simulink model "testEmplanner_cs"  (R2021b)
settings: Solver=ode5  StartTime=0.0  StopTime=60  FixedStep=1/1000  RelTol=1e-3
PreLoadFcn:
  | mbxruntime.callbacks.PreLoadFcn(bdroot);
PostLoadFcn:
  | mbxruntime.callbacks.PostLoadFcn(bdroot);
InitFcn:
  | mbxruntime.callbacks.InitFcn(bdroot);
StartFcn:
  | mbxruntime.callbacks.StartFcn(bdroot);
StopFcn:
  | mbxruntime.callbacks.StopFcn(bdroot);
model workspace (MAT data in the model file):
  mbox_table : object (value not decoded)
  model_closed = 0
  sim_status = 0
values from neighbouring files (symbols this model uses):
  c_factor = 43.75    [emplanner_init.m]
  cf = -175016    [emplanner_init.m]
  cr = -130634    [emplanner_init.m]
  global_path_x = [-1.1448 -0.145417744933 0.852705365581 1.84955224935 2.84511712279 3.83939835808 4.83239585569 5.82411007764 6.81454169183 7.80369144113 8.79156009523 9.77814843293 ... (3001 elements, 3001x1)]    [global_path.mat]
  global_path_y = [14.6488 14.6488 14.6488 14.6488 14.6488 14.6488 14.6488 14.6488 14.6488 14.6488 14.6488 14.6488 ... (3001 elements, 3001x1)]    [global_path.mat]
  KD_PID_distance = 0.0    (= 0)    [emplanner_init.m]
  KD_PID_speed = 0    [emplanner_init.m]
  KI_PID_distance = 0.0    (= 0)    [emplanner_init.m]
  KI_PID_speed = 0    [emplanner_init.m]
  KP_PID_distance = 0.5    [emplanner_init.m]
  KP_PID_speed = 1.8    [emplanner_init.m]
  la = 1.265    [emplanner_init.m]
  lb = 2.947-1.265    (= 1.682)    [emplanner_init.m]
  LQR_K1 = k(:,1)'    [emplanner_init.m]
  LQR_K2 = k(:,2)'    [emplanner_init.m]
  LQR_K3 = k(:,3)'    [emplanner_init.m]
  LQR_K4 = k(:,4)'    [emplanner_init.m]
  m = 2020    [emplanner_init.m]
  rack_displacement = [-39.14 , -37.2 , -35.29 , -33.43 , -31.6 , -29.81 , -28.06 , -26.34 , -24.66 ,      -23.01 , -21.38 , -19.79 , -18.23 , -16.69 , -15.18 , -13.7 , -12.23 , -10.8 , -9.38 , -7.98 ,     -6.61 , -5.25 , -3.91 , -2.59 , -1.29 , 0 , 1.27 , 2.54 , 3.78 , 5.02 , 6.24 , 7.46 , 8.66 ,      9.86 , 11.05 , 12.24 , 13.41 , 14.59 , 15.76 , 16.92 , 18.09 , 19.25 , 20.42 , 21.59 , 22.76 ,      23.93 , 25.11 , 26 ...(+26 chars)    [emplanner_init.m]
  right_wheel_ground = [-70 ,-67.2 , -64.4 , -61.6 , -58.8 , -56 , -53.2 , -50.4 , -47.6 , -44.8 , -42 ,      -39.2 , -36.4 , -33.6 , -30.8 , -28 , -25.2 , -22.4 , -19.6 , -16.8 , -14 , -11.2 , -8.4 , -5.6 ,      -2.8 , 0 , 2.8 , 5.6 , 8.4 , 11.2 , 14 , 16.8 , 19.6 , 22.4 , 25.2 , 28 , 30.8 , 33.6 , 36.4 ,      39.2 , 42 , 44.8 , 47.6 , 50.4 , 53.2 , 56 , 58.8 , 61.6 , 64.4 , 67.2 , 70 ]    [emplanner_init.m]
  vx_break_point = zeros(1,5000)    [emplanner_init.m]
undefined symbols (not defined in the file or in its folder): aubr, DiscIntNeverNeededParam, tablebr, vubr, warningInitialVelocity, x0
libraries: simulink x19, PreScanSimulinkLibrary x17, simulink_extras x6, Solver_SF x1
(part 4 of 14)

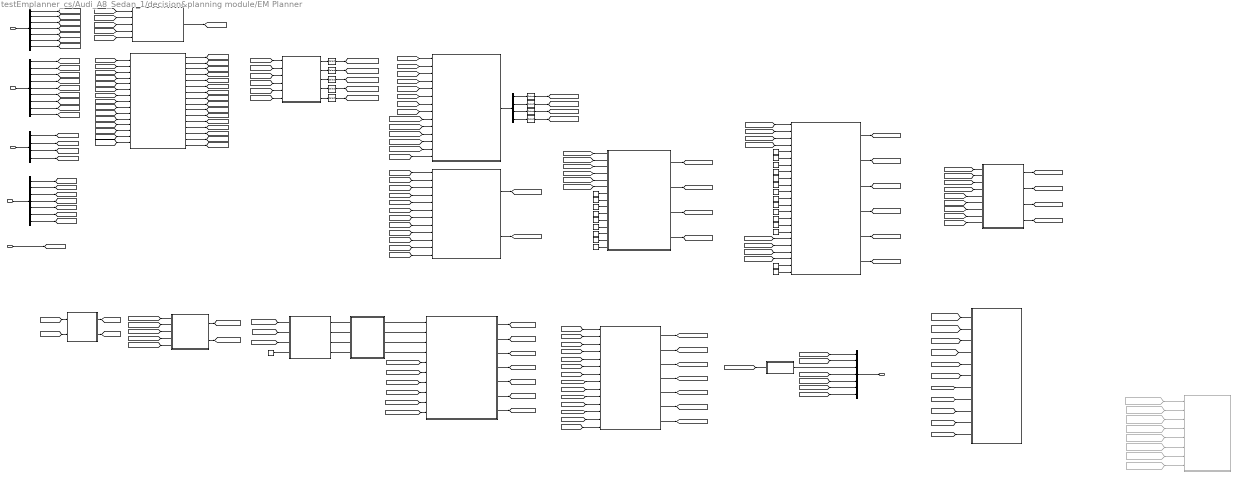
== system testEmplanner_cs/Audi_A8_Sedan_1/decision&planning module/EM Planner ==
  referenceline info : Inport
  location info : Inport  Port=2
  perception info : Inport  Port=3
  pre_planning info : Inport  Port=4
  current time : Inport  Port=5
  Bus Creator : BusCreator  Inputs=7
  Bus Selector : BusSelector  OutputSignals=host_x,host_y,host_heading_xy,host_vx,host_vy,host_yawrate,host_speed,host_ax,host_ay
  Bus Selector1 : BusSelector  OutputSignals=referenceline_x,referenceline_y,referenceline_heading,referenceline_kappa,origin_match_point_index,origin_x,origin_y
  Bus Selector2 : BusSelector  OutputSignals=obs_x_set_gcs,obs_y_set_gcs,obs_velocity_set_gcs,obs_heading_set_gcs
  Bus Selector3 : BusSelector  OutputSignals=trajectory_x_gcs,trajectory_y_gcs,trajectory_heading_gcs,trajectory_kappa_gcs,trajectory_speed_gcs,trajectory_accel_gcs,trajectory_time_gcs
  Bus Selector4 : BusSelector  OutputSignals=s_set,l_set,dl_set,ddl_set
  Cartesian2Frenet : Subsystem
  Constant : Constant  Value=1e8
  Constant1 : Constant  Value=300
  Constant10 : Constant  Value=5
  Constant11 : Constant  Value=2
  Constant12 : Constant  Value=0.1
  Constant13 : Constant  Value=0.02
  Constant14 : Constant  Value=2
  Constant15 : Constant  Value=25000
  Constant16 : Constant  Value=50
  Constant17 : Constant  Value=20
  Constant18 : Constant  Value=40
  Constant{7,19..21} (4 alike) : Constant  Value=15
  Constant2 : Constant  Value=10000
  Constant22 : Constant  Value=3
  Constant23 : Constant  Value=3
  Constant25 : Constant  Value=1.63
  Constant3 : Constant  Value=2000
  Constant4 : Constant  Value=20
  Constant5 : Constant  Value=9
  Constant6 : Constant  Value=4
  Constant8 : Constant
  Constant9 : Constant  Value=6
  Frenet2Cartesian : MATLAB Function  TreatAsAtomicUnit=on
  From165 : From  Commented=on  GotoTag=obs_st_s_in_set
  From166 : From  Commented=on  GotoTag=obs_st_s_out_set
  From167 : From  Commented=on  GotoTag=obs_st_t_in_set
  From168 : From  Commented=on  GotoTag=obs_st_t_out_set
  From177 : From  Commented=on  GotoTag=qp_s_init
  From178 : From  Commented=on  GotoTag=relative_time_init
  From90 : From  Commented=on  GotoTag=dp_speed_s
  From91 : From  Commented=on  GotoTag=dp_speed_t
  MATLAB Function : MATLAB Function  TreatAsAtomicUnit=on
  MATLAB Function3 : MATLAB Function  Commented=on  TreatAsAtomicUnit=on
  MATLAB Function5 : MATLAB Function  TreatAsAtomicUnit=on
  Selector{1..9} (9 alike) : Selector  InputPortWidth=128  IndexOptions=Index vector (dialog)  Indices=1  OutputSizes=1
  calc path length and map between point and s : MATLAB Function  TreatAsAtomicUnit=on
  calc plan start info gcs : MATLAB Function  TreatAsAtomicUnit=on
  calc speed planning start condition : MATLAB Function  TreatAsAtomicUnit=on
  decesion task : Subsystem
  genrate index to s : MATLAB Function  TreatAsAtomicUnit=on
  increase st point count : MATLAB Function  TreatAsAtomicUnit=on
  obs : Subsystem
  path and speed merge : MATLAB Function  TreatAsAtomicUnit=on
  path planning task : Subsystem
  plot : MATLAB Function  TreatAsAtomicUnit=on
  simple speed qp planning : MATLAB Function  TreatAsAtomicUnit=on
  stitch trajectory : MATLAB Function  TreatAsAtomicUnit=on
  EM Planner result : Outport
  wires:
  Bus Selector1/3 -> [referenceline_heading]  "<referenceline_heading>"
  Bus Selector1/2 -> [referenceline_y]  "<referenceline_y>"
  Bus Selector1/1 -> [referenceline_x]  "<referenceline_x>"
  referenceline info/1 -> Bus Selector1/1
  Bus Selector1/4 -> [referenceline_kappa]  "<referenceline_kappa>"
  location info/1 -> Bus Selector/1
  Bus Selector/1 -> [host_x]  "<host_x>"
  Bus Selector/2 -> [host_y]  "<host_y>"
  Bus Selector/3 -> [host_heading_xy]  "<host_heading_xy>"
  Bus Selector/4 -> [host_vx_vcs]  "<host_vx>"
  Bus Selector/5 -> [host_vy_vcs]  "<host_vy>"
  Bus Selector/6 -> [host_yawrate]  "<host_yawrate>"
  Bus Selector/7 -> [host_speed]  "<host_speed>"
  Bus Selector/8 -> [host_ax_vcs]  "<host_ax>"
  Bus Selector/9 -> [host_ay_vcs]  "<host_ay>"
  perception info/1 -> Bus Selector2/1
  Bus Selector2/1 -> [obs_x_set_gcs]  "<obs_x_set_gcs>"
  Bus Selector2/2 -> [obs_y_set_gcs]  "<obs_y_set_gcs>"
  Bus Selector2/3 -> [obs_velocity_set_gcs]  "<obs_velocity_set_gcs>"
  Bus Selector2/4 -> [obs_heading_set_gcs]  "<obs_heading_set_gcs>"
  pre_planning info/1 -> Bus Selector3/1
  Bus Selector3/1 -> [pre_trajectory_x_gcs]  "<trajectory_x_gcs>"
  Bus Selector3/2 -> [pre_trajectory_y_gcs]  "<trajectory_y_gcs>"
  Bus Selector3/3 -> [pre_trajectory_heading_gcs]  "<trajectory_heading_gcs>"
  Bus Selector3/4 -> [pre_trajectory_kappa_gcs]  "<trajectory_kappa_gcs>"
  Bus Selector3/5 -> [pre_trajectory_speed_gcs]  "<trajectory_speed_gcs>"
  Bus Selector3/6 -> [pre_trajectory_accel_gcs]  "<trajectory_accel_gcs>"
  Bus Selector3/7 -> [pre_trajectory_time]  "<trajectory_time_gcs>"
  current time/1 -> [current_time]  "current_time"
  [pre_trajectory_x_gcs] -> calc plan start info gcs/1(pre_trajectory_x)
  [pre_trajectory_y_gcs] -> calc plan start info gcs/2(pre_trajectory_y)
  [pre_trajectory_heading_gcs] -> calc plan start info gcs/3(pre_trajectory_heading)
  [pre_trajectory_kappa_gcs] -> calc plan start info gcs/4(pre_trajectory_kappa)
  [pre_trajectory_speed_gcs] -> calc plan start info gcs/5(pre_trajectory_velocity)
  [pre_trajectory_accel_gcs] -> calc plan start info gcs/6(pre_trajectory_accel)
  [pre_trajectory_time] -> calc plan start info gcs/7(pre_trajectory_time)
  [current_time] -> calc plan start info gcs/8(current_time)
  [host_x] -> calc plan start info gcs/9(host_x)
  [host_y] -> calc plan start info gcs/10(host_y)
  [host_heading_xy] -> calc plan start info gcs/11(host_heading_xy)
  [host_vx_vcs] -> calc plan start info gcs/12(host_vx)
  [host_vy_vcs] -> calc plan start info gcs/13(host_vy)
  [host_ay_vcs] -> calc plan start info gcs/15(host_ay)
  [host_ax_vcs] -> calc plan start info gcs/14(host_ax)
  calc plan start info gcs/16(stitch_time) -> [stitch_time]
  calc plan start info gcs/15(stitch_accel) -> [stitch_accel_gcs]
  calc plan start info gcs/14(stitch_speed) -> [stitch_speed_gcs]
  calc plan start info gcs/13(stitch_kappa) -> [stitch_kappa_gcs]
  calc plan start info gcs/12(stitch_heading) -> [stitch_heading_gcs]
  calc plan start info gcs/11(stitch_y) -> [stitch_y_gcs]
  calc plan start info gcs/10(stitch_x) -> [stitch_x_gcs]
  calc plan start info gcs/9(plan_start_time) -> [plan_start_time]
  calc plan start info gcs/8(plan_start_ay) -> [plan_start_ay_gcs]
  calc plan start info gcs/7(plan_start_ax) -> [plan_start_ax_gcs]
  calc plan start info gcs/6(plan_start_vy) -> [plan_start_vy_gcs]
  calc plan start info gcs/5(plan_start_vx) -> [plan_start_vx_gcs]
  calc plan start info gcs/4(plan_start_kappa) -> [plan_start_kappa_gcs]
  calc plan start info gcs/1(plan_start_x) -> [plan_start_x_gcs]
  calc plan start info gcs/2(plan_start_y) -> [plan_start_y_gcs]
  calc plan start info gcs/3(plan_start_heading) -> [plan_start_heading_gcs]
  Bus Selector1/5 -> [origin_match_point_index]  "<origin_match_point_index>"
  Bus Selector1/6 -> [origin_x]  "<origin_x>"
  Bus Selector1/7 -> [origin_y]  "<origin_y>"
  [referenceline_x] -> genrate index to s/1(path_x)
  [referenceline_y] -> genrate index to s/2(path_y)
  [origin_x] -> genrate index to s/3(origin_x)
  [origin_y] -> genrate index to s/4(origin_y)
  [origin_match_point_index] -> genrate index to s/5(origin_match_point_index)
  genrate index to s/1(index2s) -> [index2s]
  [referenceline_y] -> MATLAB Function5/4(frenet_path_y)
  Selector4/1 -> [plan_start_proj_heading]
  Selector1/1 -> [plan_start_match_point_index]
  [referenceline_x] -> MATLAB Function5/3(frenet_path_x)
  MATLAB Function5/2(proj_x_set) -> Selector2/1
  [plan_start_x_gcs] -> MATLAB Function5/1(x_set)
  [plan_start_y_gcs] -> MATLAB Function5/2(y_set)
  MATLAB Function5/1(match_point_index_set) -> Selector1/1
  [referenceline_heading] -> MATLAB Function5/5(frenet_path_heading)
  Selector2/1 -> [plan_start_proj_x]
  [referenceline_kappa] -> MATLAB Function5/6(frenet_path_kappa)
  MATLAB Function5/3(proj_y_set) -> Selector3/1
  MATLAB Function5/4(proj_heading_set) -> Selector4/1
  MATLAB Function5/5(proj_kappa_set) -> Selector5/1
  Selector5/1 -> [plan_start_proj_kappa]
  Selector3/1 -> [plan_start_proj_y]
  [plan_start_x_gcs] -> Cartesian2Frenet/1(x_set)
  [plan_start_y_gcs] -> Cartesian2Frenet/2(y_set)
  [plan_start_vx_gcs] -> Cartesian2Frenet/3(vx_set)
  [plan_start_vy_gcs] -> Cartesian2Frenet/4(vy_set)
  [plan_start_ax_gcs] -> Cartesian2Frenet/5(ax_set)
  [plan_start_ay_gcs] -> Cartesian2Frenet/6(ay_set)
  [referenceline_x] -> Cartesian2Frenet/7(frenet_path_x)
  [referenceline_y] -> Cartesian2Frenet/8(frenet_path_y)
  [plan_start_match_point_index] -> Cartesian2Frenet/9(proj_match_point_index_set)
  [plan_start_proj_x] -> Cartesian2Frenet/10(proj_x_set)
  [plan_start_proj_y] -> Cartesian2Frenet/11(proj_y_set)
  [plan_start_proj_heading] -> Cartesian2Frenet/12(proj_heading_set)
  [plan_start_proj_kappa] -> Cartesian2Frenet/13(proj_kappa_set)
  [index2s] -> Cartesian2Frenet/14(index2s)
  Cartesian2Frenet/1(Cartesian2FrenetOut) -> Bus Selector4/1
  Bus Selector4/1 -> Selector6/1  "<s_set>"
  Bus Selector4/2 -> Selector7/1  "<l_set>"
  Bus Selector4/3 -> Selector9/1  "<dl_set>"
  Bus Selector4/4 -> Selector8/1  "<ddl_set>"
  Selector6/1 -> [plan_start_s]
  Selector9/1 -> [plan_start_dl]
  Selector7/1 -> [plan_start_l]
  Selector8/1 -> [plan_start_ddl]
  [host_x] -> obs/1(host_x)
  [host_y] -> obs/2(host_y)
  [host_heading_xy] -> obs/3(host_heading_xy)
  [obs_x_set_gcs] -> obs/4(obs_x_set_gcs)
  [obs_y_set_gcs] -> obs/5(obs_y_set_gcs)
  [obs_velocity_set_gcs] -> obs/6(obs_velocity_set_gcs)
  [obs_heading_set_gcs] -> obs/7(obs_heading_set_gcs)
  [referenceline_y] -> obs/9(referenceline_y)
  [referenceline_heading] -> obs/10(referenceline_heading)
  [referenceline_kappa] -> obs/11(referenceline_kappa)
  [index2s] -> obs/12(index2s)
  [referenceline_x] -> obs/8(referenceline_x)
  obs/1(static_obs_s_set) -> [static_obs_s_set]
  obs/2(static_obs_l_set) -> [static_obs_l_set]
  [qp_path_s] -> Frenet2Cartesian/1(s_set)
  [qp_path_l] -> Frenet2Cartesian/2(l_set)
  [qp_path_dl] -> Frenet2Cartesian/3(dl_set)
  [qp_path_ddl] -> Frenet2Cartesian/4(ddl_set)
  [referenceline_x] -> Frenet2Cartesian/5(frenet_path_x)
  [referenceline_y] -> Frenet2Cartesian/6(frenet_path_y)
  [referenceline_heading] -> Frenet2Cartesian/7(frenet_path_heading)
  [referenceline_kappa] -> Frenet2Cartesian/8(frenet_path_kappa)
  [index2s] -> Frenet2Cartesian/9(index2s)
  Frenet2Cartesian/3(heading_set) -> [trajectory_heading_init]
  Frenet2Cartesian/4(kappa_set) -> [trajectory_kappa_init]
  Frenet2Cartesian/2(y_set) -> [trajectory_y_init]
  Frenet2Cartesian/1(x_set) -> [trajectory_x_init]
  Constant9/1 -> simple speed qp planning/4(recommend_T)
  [trajectory_speed_final] -> Bus Creator/5  "trajectory_speed_gcs"
  [stitch_heading_gcs] -> stitch trajectory/10(stitch_heading)
  [trajectory_x_final] -> Bus Creator/1  "trajectory_x_gcs"
  [trajectory_accel] -> stitch trajectory/6(trajectory_accel)
  [plan_start_s_dot2] -> simple speed qp planning/2(plan_start_s_dot2)
  [stitch_time] -> stitch trajectory/14(stitch_time)
  [plan_start_vy_gcs] -> calc speed planning start condition/2(plan_start_vy)
  [stitch_x_gcs] -> stitch trajectory/8(stitch_x)
  path and speed merge/7(trajectory_time) -> [trajectory_time]
  path and speed merge/5(trajectory_speed) -> [trajectory_speed]
  [trajectory_speed] -> stitch trajectory/5(trajectory_speed)
  stitch trajectory/2(trajectory_y_final) -> [trajectory_y_final]
  [path_s] -> path and speed merge/6(path_s)
  [plan_start_time] -> path and speed merge/5(current_time)
  [stitch_kappa_gcs] -> stitch trajectory/11(stitch_kappa)
  [plan_start_ax_gcs] -> calc speed planning start condition/3(plan_start_ax)
  path and speed merge/4(trajectory_kappa) -> [trajectory_kappa]
  calc speed planning start condition/1(plan_start_s_dot) -> [plan_start_s_dot]
  path and speed merge/2(trajectory_y) -> [trajectory_y]
  [plan_start_ay_gcs] -> calc speed planning start condition/4(plan_start_ay)
  stitch trajectory/6(trajectory_accel_final) -> [trajectory_accel_final]
  stitch trajectory/1(trajectory_x_final) -> [trajectory_x_final]
  [trajectory_y_init] -> calc path length and map between point and s/2(trajectory_y)
  [trajectory_accel_final] -> Bus Creator/6  "trajectory_accel_gcs"
  calc path length and map between point and s/2(path_s) -> [path_s]
  [stitch_y_gcs] -> stitch trajectory/9(stitch_y)
  [trajectory_kappa] -> stitch trajectory/4(trajectory_kappa)
  [trajectory_kappa_final] -> Bus Creator/4  "trajectory_kappa_gcs"
  stitch trajectory/3(trajectory_heading_final) -> [trajectory_heading_final]
  increase st point count/2(s_dot) -> path and speed merge/2(s_dot)
  [plan_start_heading_gcs] -> calc speed planning start condition/5(plan_start_heading)
  [trajectory_x_init] -> path and speed merge/7(trajectory_x_init)
  calc path length and map between point and s/1(path_s_end) -> [path_s_end]
  increase st point count/3(s_dot2) -> path and speed merge/3(s_dot2)
  increase st point count/1(s) -> path and speed merge/1(s)
  [trajectory_y] -> stitch trajectory/2(trajectory_y)
  [trajectory_kappa_init] -> path and speed merge/10(trajectory_kappa_init)
  [stitch_accel_gcs] -> stitch trajectory/13(stitch_accel)
  simple speed qp planning/3(s_dot2_init) -> increase st point count/3(s_dot2_init)
  simple speed qp planning/2(s_dot_init) -> increase st point count/2(s_dot_init)
  [trajectory_y_init] -> path and speed merge/8(trajectory_y_init)
  MATLAB Function/1(y) -> Bus Creator/3  "trajectory_heading_gcs"
  calc speed planning start condition/2(plan_start_s_dot2) -> [plan_start_s_dot2]
  [trajectory_heading_init] -> path and speed merge/9(trajectory_heading_init)
  [trajectory_x_init] -> calc path length and map between point and s/1(trajectory_x)
  [trajectory_heading] -> stitch trajectory/3(trajectory_heading)
  [trajectory_time] -> stitch trajectory/7(trajectory_time)
  [trajectory_x] -> stitch trajectory/1(trajectory_x)
  increase st point count/4(relative_time) -> path and speed merge/4(relative_time)
  path and speed merge/6(trajectory_accel) -> [trajectory_accel]
  path and speed merge/3(trajectory_heading) -> [trajectory_heading]
  stitch trajectory/4(trajectory_kappa_final) -> [trajectory_kappa_final]
  simple speed qp planning/4(relative_time_init) -> increase st point count/4(relative_time_init)
  stitch trajectory/5(trajectory_speed_final) -> [trajectory_speed_final]
  [plan_start_s_dot] -> simple speed qp planning/1(plan_start_s_dot)
  [path_s_end] -> simple speed qp planning/3(s_end)
  [trajectory_y_final] -> Bus Creator/2  "trajectory_y_gcs"
  simple speed qp planning/1(s_init) -> increase st point count/1(s_init)
  [trajectory_time_final] -> Bus Creator/7  "trajectory_time_gcs"
  Bus Creator/1 -> EM Planner result/1
  [stitch_speed_gcs] -> stitch trajectory/12(stitch_speed)
  path and speed merge/1(trajectory_x) -> [trajectory_x]
  stitch trajectory/7(trajectory_time_final) -> [trajectory_time_final]
  [plan_start_vx_gcs] -> calc speed planning start condition/1(plan_start_vx)
  [static_obs_s_set] -> plot/7(obs_s_set)
  [dp_path_l_final] -> plot/2(dp_l)
  [static_obs_l_set] -> plot/8(obs_l_set)
  [plan_start_dl] -> plot/11(start_dl)
  [qp_path_l] -> plot/4(qp_l)
  [plan_start_s] -> plot/9(start_s)
  [plan_start_l] -> plot/10(start_l)
  [dp_path_s_final] -> plot/1(dp_s)
  From168/1 -> MATLAB Function3/8(obs_t_out_set)
  From90/1 -> MATLAB Function3/1(dp_speed_s)
  From178/1 -> MATLAB Function3/4(qp_speed_t)
  From166/1 -> MATLAB Function3/6(obs_s_out_set)
  From177/1 -> MATLAB Function3/3(qp_speed_s)
  From167/1 -> MATLAB Function3/7(obs_t_in_set)
  From165/1 -> MATLAB Function3/5(obs_s_in_set)
  From91/1 -> MATLAB Function3/2(dp_speed_t)
  [l_min] -> plot/5(l_min)
  [l_max] -> plot/6(l_max)
  [qp_path_s] -> plot/3(qp_s)
  [dp_path_s_final] -> path planning task/1(dp_path_s)
  [dp_path_l_final] -> path planning task/2(dp_path_l)
  [static_obs_s_set] -> path planning task/3(static_obs_s_set)
  [static_obs_l_set] -> path planning task/4(static_obs_l_set)
  Constant10/1 -> path planning task/5(static_obs_length)
  Constant11/1 -> path planning task/6(static_obs_width)
  Constant14/1 -> path planning task/7(qp_cost_l)
  Constant15/1 -> path planning task/8(qp_cost_dl)
  Constant16/1 -> path planning task/9(qp_cost_ddl)
  Constant17/1 -> path planning task/10(qp_cost_dddl)
  Constant18/1 -> path planning task/11(qp_cost_centre)
  Constant19/1 -> path planning task/12(qp_cost_end_l)
  Constant20/1 -> path planning task/13(qp_cost_end_dl)
  Constant21/1 -> path planning task/14(qp_cost_end_ddl)
  Constant22/1 -> path planning task/15(host_d1)
  Constant23/1 -> path planning task/16(host_d2)
  Constant25/1 -> path planning task/17(host_w)
  [plan_start_s] -> path planning task/18(plan_start_s)
  [plan_start_l] -> path planning task/19(plan_start_l)
  [plan_start_dl] -> path planning task/20(plan_start_dl)
  [plan_start_ddl] -> path planning task/21(plan_start_ddl)
  Constant12/1 -> path planning task/22(delta_dl_max)
  Constant13/1 -> path planning task/23(delta_ddl_max)
  path planning task/1(qp_path_s) -> [qp_path_s]
  path planning task/2(qp_path_l) -> [qp_path_l]
  path planning task/3(qp_path_dl) -> [qp_path_dl]
  path planning task/4(qp_path_ddl) -> [qp_path_ddl]
  [static_obs_s_set] -> decesion task/1(obs_s_set)
  [static_obs_l_set] -> decesion task/2(obs_l_set)
  [plan_start_s] -> decesion task/3(plan_start_s)
  [plan_start_l] -> decesion task/4(plan_start_l)
  [plan_start_dl] -> decesion task/5(plan_start_dl)
  [plan_start_ddl] -> decesion task/6(plan_start_dll)
  Constant/1 -> decesion task/7(dp_cost_collision)
  Constant1/1 -> decesion task/8(dp_cost_smooth_dl)
  Constant3/1 -> decesion task/9(dp_cost_smooth_ddl)
  Constant2/1 -> decesion task/10(dp_cost_smooth_dddl)
  Constant4/1 -> decesion task/11(dp_cost_ref)
  Constant5/1 -> decesion task/12(dp_row)
  Constant6/1 -> decesion task/13(dp_col)
  Constant7/1 -> decesion task/14(dp_sample_s)
  Constant8/1 -> decesion task/15(dp_sample_l)
  decesion task/1(dp_path_s_final) -> [dp_path_s_final]
  decesion task/2(dp_path_l_final) -> [dp_path_l_final]
  decesion task/3(dp_path_dl_final) -> [dp_path_dl_final]
  decesion task/4(dp_path_ddl_final) -> [dp_path_ddl_final]
  path planning task/6(qp_l_max) -> [l_max]
  path planning task/5(qp_l_min) -> [l_min]
  [trajectory_heading_final] -> MATLAB Function/1(trajectory_heading_final)

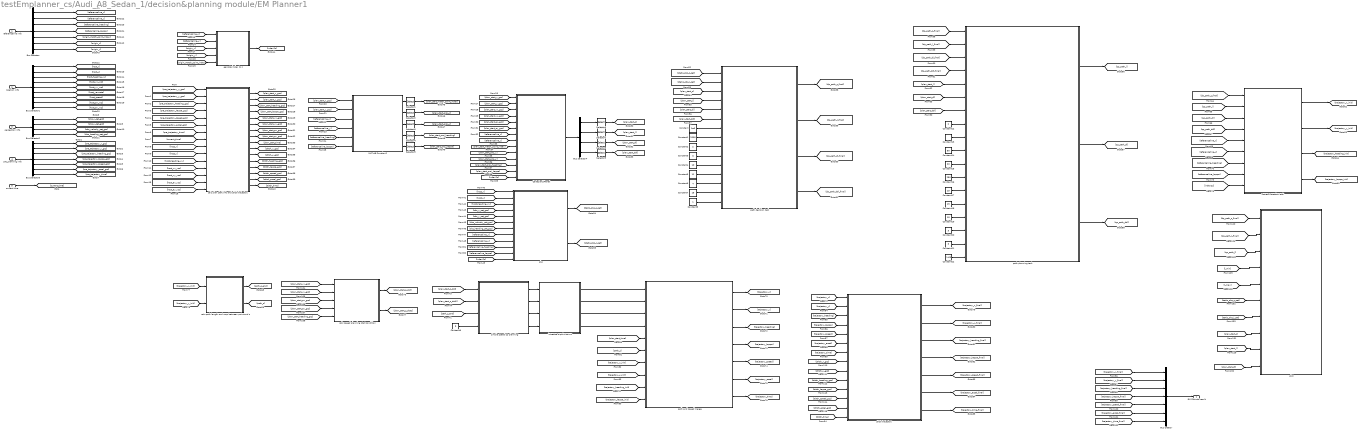
== system testEmplanner_cs/Audi_A8_Sedan_1/decision&planning module/EM Planner1 ==
  referenceline info : Inport
  location info : Inport  Port=2
  perception info : Inport  Port=3
  pre_planning info : Inport  Port=4
  current time : Inport  Port=5
  Bus Creator : BusCreator  Inputs=7
  Bus Selector : BusSelector  OutputSignals=referenceline_x,referenceline_y,referenceline_heading,referenceline_kappa,origin_match_point_index,origin_x,origin_y
  Bus Selector1 : BusSelector  OutputSignals=host_x,host_y,host_heading_xy,host_vx,host_vy,host_yawrate,host_speed,host_ax,host_ay
  Bus Selector2 : BusSelector  OutputSignals=obs_x_set_gcs,obs_y_set_gcs,obs_velocity_set_gcs,obs_heading_set_gcs
  Bus Selector3 : BusSelector  OutputSignals=trajectory_x_gcs,trajectory_y_gcs,trajectory_heading_gcs,trajectory_kappa_gcs,trajectory_speed_gcs,trajectory_accel_gcs,trajectory_time_gcs
  Bus Selector4 : BusSelector  OutputSignals=s_set,l_set,dl_set,ddl_set
  Cartesian2Frenet : Subsystem
  Constant : Constant  Value=1e6
  Constant1 : Constant  Value=2000
  Constant12 : Constant  Value=2
  Constant13 : Constant  Value=25000
  Constant14 : Constant  Value=50
  Constant15 : Constant  Value=20
  Constant16 : Constant  Value=250
  Constant{7,17..19} (4 alike) : Constant  Value=15
  Constant2 : Constant  Value=2
  Constant20 : Constant  Value=3
  Constant21 : Constant  Value=3
  Constant22 : Constant  Value=1.63
  Constant3 : Constant  Value=3
  Constant4 : Constant  Value=10
  Constant5 : Constant  Value=11
  Constant6 : Constant  Value=4
  Constant8 : Constant
  Constant9 : Constant  Value=6
  Frenet2Cartesian task : MATLAB Function  TreatAsAtomicUnit=on
  MATLAB Function2 : MATLAB Function  TreatAsAtomicUnit=on
  Selector{1..9} (9 alike) : Selector  InputPortWidth=128  IndexOptions=Index vector (dialog)  Indices=1  OutputSizes=1
  calc path length and map between point and s : MATLAB Function  TreatAsAtomicUnit=on
  calc plan start info and stitch trajectory : MATLAB Function  TreatAsAtomicUnit=on
  calc speed planning start condition : MATLAB Function  TreatAsAtomicUnit=on
  genrate index to s : MATLAB Function  TreatAsAtomicUnit=on
  increase st point count : MATLAB Function  TreatAsAtomicUnit=on
  obs : Subsystem
  path and speed merge : MATLAB Function  TreatAsAtomicUnit=on
  path decision task : Subsystem
  path planning task : Subsystem
  plot : MATLAB Function  TreatAsAtomicUnit=on
  simple speed qp planning : MATLAB Function  TreatAsAtomicUnit=on
  stitch trajectory : MATLAB Function  TreatAsAtomicUnit=on
  EM Planner result : Outport
  wires:
  referenceline info/1 -> Bus Selector/1
  location info/1 -> Bus Selector1/1
  perception info/1 -> Bus Selector2/1
  pre_planning info/1 -> Bus Selector3/1
  current time/1 -> [current_time]
  Bus Selector3/1 -> [pre_trajectory_x_gcs]  "<trajectory_x_gcs>"
  Bus Selector3/2 -> [pre_trajectory_y_gcs]  "<trajectory_y_gcs>"
  Bus Selector3/3 -> [pre_trajectory_heading_gcs]  "<trajectory_heading_gcs>"
  Bus Selector3/4 -> [pre_trajectory_kappa_gcs]  "<trajectory_kappa_gcs>"
  Bus Selector3/5 -> [pre_trajectory_speed_gcs]  "<trajectory_speed_gcs>"
  Bus Selector3/6 -> [pre_trajectory_accel_gcs]  "<trajectory_accel_gcs>"
  Bus Selector3/7 -> [pre_trajectory_time]  "<trajectory_time_gcs>"
  Bus Selector2/1 -> [obs_x_set_gcs]  "<obs_x_set_gcs>"
  Bus Selector2/2 -> [obs_y_set_gcs]  "<obs_y_set_gcs>"
  Bus Selector2/3 -> [obs_velocity_set_gcs]  "<obs_velocity_set_gcs>"
  Bus Selector2/4 -> [obs_heading_set_gcs]  "<obs_heading_set_gcs>"
  Bus Selector1/1 -> [host_x]  "<host_x>"
  Bus Selector1/2 -> [host_y]  "<host_y>"
  Bus Selector1/3 -> [host_heading_xy]  "<host_heading_xy>"
  Bus Selector1/4 -> [host_vx_vcs]  "<host_vx>"
  Bus Selector1/5 -> [host_vy_vcs]  "<host_vy>"
  Bus Selector1/6 -> [host_yawrate]  "<host_yawrate>"
  Bus Selector1/7 -> [host_speed]  "<host_speed>"
  Bus Selector1/8 -> [host_ax_vcs]  "<host_ax>"
  Bus Selector1/9 -> [host_ay_vcs]  "<host_ay>"
  Bus Selector/1 -> [referenceline_x]  "<referenceline_x>"
  Bus Selector/2 -> [referenceline_y]  "<referenceline_y>"
  Bus Selector/3 -> [referenceline_heading]  "<referenceline_heading>"
  Bus Selector/4 -> [referenceline_kappa]  "<referenceline_kappa>"
  [host_ay_vcs] -> calc plan start info and stitch trajectory/15(host_ay)
  [host_ax_vcs] -> calc plan start info and stitch trajectory/14(host_ax)
  [host_vy_vcs] -> calc plan start info and stitch trajectory/13(host_vy)
  [host_vx_vcs] -> calc plan start info and stitch trajectory/12(host_vx)
  [host_heading_xy] -> calc plan start info and stitch trajectory/11(host_heading_xy)
  [host_y] -> calc plan start info and stitch trajectory/10(host_y)
  [host_x] -> calc plan start info and stitch trajectory/9(host_x)
  [current_time] -> calc plan start info and stitch trajectory/8(current_time)
  [pre_trajectory_x_gcs] -> calc plan start info and stitch trajectory/1(pre_trajectory_x)
  [pre_trajectory_y_gcs] -> calc plan start info and stitch trajectory/2(pre_trajectory_y)
  [pre_trajectory_time] -> calc plan start info and stitch trajectory/7(pre_trajectory_time)
  [pre_trajectory_accel_gcs] -> calc plan start info and stitch trajectory/6(pre_trajectory_accel)
  [pre_trajectory_speed_gcs] -> calc plan start info and stitch trajectory/5(pre_trajectory_velocity)
  [pre_trajectory_kappa_gcs] -> calc plan start info and stitch trajectory/4(pre_trajectory_kappa)
  [pre_trajectory_heading_gcs] -> calc plan start info and stitch trajectory/3(pre_trajectory_heading)
  calc plan start info and stitch trajectory/1(plan_start_x) -> [plan_start_x_gcs]
  calc plan start info and stitch trajectory/2(plan_start_y) -> [plan_start_y_gcs]
  calc plan start info and stitch trajectory/3(plan_start_heading) -> [plan_start_heading_gcs]
  calc plan start info and stitch trajectory/4(plan_start_kappa) -> [plan_start_kappa_gcs]
  calc plan start info and stitch trajectory/5(plan_start_vx) -> [plan_start_vx_gcs]
  calc plan start info and stitch trajectory/6(plan_start_vy) -> [plan_start_vy_gcs]
  calc plan start info and stitch trajectory/7(plan_start_ax) -> [plan_start_ax_gcs]
  calc plan start info and stitch trajectory/8(plan_start_ay) -> [plan_start_ay_gcs]
  calc plan start info and stitch trajectory/9(plan_start_time) -> [plan_start_time]
  calc plan start info and stitch trajectory/10(stitch_x) -> [stitch_x_gcs]
  calc plan start info and stitch trajectory/11(stitch_y) -> [stitch_y_gcs]
  calc plan start info and stitch trajectory/12(stitch_heading) -> [stitch_heading_gcs]
  calc plan start info and stitch trajectory/13(stitch_kappa) -> [stitch_kappa_gcs]
  calc plan start info and stitch trajectory/14(stitch_speed) -> [stitch_speed_gcs]
  calc plan start info and stitch trajectory/15(stitch_accel) -> [stitch_accel_gcs]
  calc plan start info and stitch trajectory/16(stitch_time) -> [stitch_time]
  Bus Selector/5 -> [origin_match_point_index]  "<origin_match_point_index>"
  Bus Selector/6 -> [origin_x]  "<origin_x>"
  Bus Selector/7 -> [origin_y]  "<origin_y>"
  [referenceline_x] -> genrate index to s/1(path_x)
  [referenceline_y] -> genrate index to s/2(path_y)
  [origin_x] -> genrate index to s/3(origin_x)
  [origin_y] -> genrate index to s/4(origin_y)
  [origin_match_point_index] -> genrate index to s/5(origin_match_point_index)
  genrate index to s/1(index2s) -> [index2s]
  MATLAB Function2/5(proj_kappa_set) -> Selector5/1
  MATLAB Function2/3(proj_y_set) -> Selector3/1
  MATLAB Function2/1(match_point_index_set) -> Selector1/1
  MATLAB Function2/4(proj_heading_set) -> Selector4/1
  MATLAB Function2/2(proj_x_set) -> Selector2/1
  [plan_start_x_gcs] -> MATLAB Function2/1(x_set)
  [plan_start_y_gcs] -> MATLAB Function2/2(y_set)
  [referenceline_x] -> MATLAB Function2/3(frenet_path_x)
  [referenceline_y] -> MATLAB Function2/4(frenet_path_y)
  [referenceline_heading] -> MATLAB Function2/5(frenet_path_heading)
  [referenceline_kappa] -> MATLAB Function2/6(frenet_path_kappa)
  Selector1/1 -> [plan_start_match_point_index]
  Selector2/1 -> [plan_start_proj_x]
  Selector3/1 -> [plan_start_proj_y]
  Selector4/1 -> [plan_start_proj_heading]
  Selector5/1 -> [plan_start_proj_kappa]
  [plan_start_y_gcs] -> Cartesian2Frenet/2(y_set)
  [plan_start_x_gcs] -> Cartesian2Frenet/1(x_set)
  [plan_start_vx_gcs] -> Cartesian2Frenet/3(vx_set)
  [plan_start_vy_gcs] -> Cartesian2Frenet/4(vy_set)
  [plan_start_ax_gcs] -> Cartesian2Frenet/5(ax_set)
  [plan_start_ay_gcs] -> Cartesian2Frenet/6(ay_set)
  [referenceline_x] -> Cartesian2Frenet/7(frenet_path_x)
  [referenceline_y] -> Cartesian2Frenet/8(frenet_path_y)
  [plan_start_match_point_index] -> Cartesian2Frenet/9(proj_match_point_index_set)
  [plan_start_proj_x] -> Cartesian2Frenet/10(proj_x_set)
  [plan_start_proj_y] -> Cartesian2Frenet/11(proj_y_set)
  [plan_start_proj_heading] -> Cartesian2Frenet/12(proj_heading_set)
  [plan_start_proj_kappa] -> Cartesian2Frenet/13(proj_kappa_set)
  Cartesian2Frenet/1(Cartesian2FrenetOut) -> Bus Selector4/1
  Bus Selector4/4 -> Selector9/1  "<ddl_set>"
  Bus Selector4/3 -> Selector8/1  "<dl_set>"
  Bus Selector4/2 -> Selector7/1  "<l_set>"
  Bus Selector4/1 -> Selector6/1  "<s_set>"
  Selector6/1 -> [plan_start_s]
  Selector7/1 -> [plan_start_l]
  Selector8/1 -> [plan_start_dl]
  Selector9/1 -> [plan_start_ddl]
  [index2s] -> Cartesian2Frenet/14(index2s)
  [host_x] -> obs/1(host_x)
  [host_y] -> obs/2(host_y)
  [host_heading_xy] -> obs/3(host_heading_xy)
  [obs_x_set_gcs] -> obs/4(obs_x_set_gcs)
  [obs_y_set_gcs] -> obs/5(obs_y_set_gcs)
  [obs_velocity_set_gcs] -> obs/6(obs_velocity_set_gcs)
  [obs_heading_set_gcs] -> obs/7(obs_heading_set_gcs)
  [referenceline_x] -> obs/8(referenceline_x)
  [referenceline_y] -> obs/9(referenceline_y)
  [referenceline_heading] -> obs/10(referenceline_heading)
  [referenceline_kappa] -> obs/11(referenceline_kappa)
  [index2s] -> obs/12(index2s)
  obs/1(static_obs_s_set) -> [static_obs_s_set]
  obs/2(static_obs_l_set) -> [static_obs_l_set]
  path and speed merge/7(trajectory_time) -> [trajectory_time]
  path and speed merge/1(trajectory_x) -> [trajectory_x]
  [trajectory_speed] -> stitch trajectory/5(trajectory_speed)
  path and speed merge/4(trajectory_kappa) -> [trajectory_kappa]
  [plan_start_vy_gcs] -> calc speed planning start condition/2(plan_start_vy)
  [stitch_time] -> stitch trajectory/14(stitch_time)
  calc path length and map between point and s/2(path_s) -> [path_s]
  [plan_start_heading_gcs] -> calc speed planning start condition/5(plan_start_heading)
  simple speed qp planning/2(s_dot_init) -> increase st point count/2(s_dot_init)
  Bus Creator/1 -> EM Planner result/1
  simple speed qp planning/1(s_init) -> increase st point count/1(s_init)
  [trajectory_x_final] -> Bus Creator/1  "trajectory_x_gcs"
  stitch trajectory/4(trajectory_kappa_final) -> [trajectory_kappa_final]
  [plan_start_ax_gcs] -> calc speed planning start condition/3(plan_start_ax)
  calc speed planning start condition/1(plan_start_s_dot) -> [plan_start_s_dot]
  [plan_start_ay_gcs] -> calc speed planning start condition/4(plan_start_ay)
  [stitch_speed_gcs] -> stitch trajectory/12(stitch_speed)
  [trajectory_time_final] -> Bus Creator/7  "trajectory_time_gcs"
  Constant9/1 -> simple speed qp planning/4(recommend_T)
  [stitch_x_gcs] -> stitch trajectory/8(stitch_x)
  stitch trajectory/1(trajectory_x_final) -> [trajectory_x_final]
  [trajectory_accel_final] -> Bus Creator/6  "trajectory_accel_gcs"
  [stitch_heading_gcs] -> stitch trajectory/10(stitch_heading)
  [trajectory_speed_final] -> Bus Creator/5  "trajectory_speed_gcs"
  [stitch_y_gcs] -> stitch trajectory/9(stitch_y)
  stitch trajectory/6(trajectory_accel_final) -> [trajectory_accel_final]
  [plan_start_s_dot2] -> simple speed qp planning/2(plan_start_s_dot2)
  increase st point count/3(s_dot2) -> path and speed merge/3(s_dot2)
  [plan_start_vx_gcs] -> calc speed planning start condition/1(plan_start_vx)
  [trajectory_heading_final] -> Bus Creator/3  "trajectory_heading_gcs"
  [trajectory_accel] -> stitch trajectory/6(trajectory_accel)
  [trajectory_kappa] -> stitch trajectory/4(trajectory_kappa)
  stitch trajectory/7(trajectory_time_final) -> [trajectory_time_final]
  [trajectory_x_init] -> path and speed merge/7(trajectory_x_init)
  stitch trajectory/2(trajectory_y_final) -> [trajectory_y_final]
  increase st point count/2(s_dot) -> path and speed merge/2(s_dot)
  stitch trajectory/3(trajectory_heading_final) -> [trajectory_heading_final]
  [trajectory_kappa_final] -> Bus Creator/4  "trajectory_kappa_gcs"
  [plan_start_s_dot] -> simple speed qp planning/1(plan_start_s_dot)
  path and speed merge/3(trajectory_heading) -> [trajectory_heading]
  simple speed qp planning/3(s_dot2_init) -> increase st point count/3(s_dot2_init)
  stitch trajectory/5(trajectory_speed_final) -> [trajectory_speed_final]
  [trajectory_y_final] -> Bus Creator/2  "trajectory_y_gcs"
  [trajectory_y] -> stitch trajectory/2(trajectory_y)
  calc path length and map between point and s/1(path_s_end) -> [path_s_end]
  calc speed planning start condition/2(plan_start_s_dot2) -> [plan_start_s_dot2]
  [trajectory_kappa_init] -> path and speed merge/10(trajectory_kappa_init)
  [stitch_accel_gcs] -> stitch trajectory/13(stitch_accel)
  increase st point count/1(s) -> path and speed merge/1(s)
  [trajectory_x] -> stitch trajectory/1(trajectory_x)
  [trajectory_y_init] -> calc path length and map between point and s/2(trajectory_y)
  [path_s_end] -> simple speed qp planning/3(s_end)
  path and speed merge/6(trajectory_accel) -> [trajectory_accel]
  [stitch_kappa_gcs] -> stitch trajectory/11(stitch_kappa)
  increase st point count/4(relative_time) -> path and speed merge/4(relative_time)
  [path_s] -> path and speed merge/6(path_s)
  path and speed merge/2(trajectory_y) -> [trajectory_y]
  [trajectory_heading_init] -> path and speed merge/9(trajectory_heading_init)
  [plan_start_time] -> path and speed merge/5(current_time)
  path and speed merge/5(trajectory_speed) -> [trajectory_speed]
  simple speed qp planning/4(relative_time_init) -> increase st point count/4(relative_time_init)
  [trajectory_y_init] -> path and speed merge/8(trajectory_y_init)
  [trajectory_time] -> stitch trajectory/7(trajectory_time)
  [trajectory_heading] -> stitch trajectory/3(trajectory_heading)
  [trajectory_x_init] -> calc path length and map between point and s/1(trajectory_x)
  [index2s] -> Frenet2Cartesian task/9(index2s)
  [referenceline_x] -> Frenet2Cartesian task/5(frenet_path_x)
  [referenceline_y] -> Frenet2Cartesian task/6(frenet_path_y)
  [referenceline_heading] -> Frenet2Cartesian task/7(frenet_path_heading)
  [referenceline_kappa] -> Frenet2Cartesian task/8(frenet_path_kappa)
  Frenet2Cartesian task/1(x_set) -> [trajectory_x_init]
  Frenet2Cartesian task/2(y_set) -> [trajectory_y_init]
  Frenet2Cartesian task/3(heading_set) -> [trajectory_heading_init]
  Frenet2Cartesian task/4(kappa_set) -> [trajectory_kappa_init]
  [qp_path_ddl] -> Frenet2Cartesian task/4(ddl_set)
  [qp_path_dl] -> Frenet2Cartesian task/3(dl_set)
  [qp_path_l] -> Frenet2Cartesian task/2(l_set)
  [dp_path_s_final] -> Frenet2Cartesian task/1(s_set)
  [qp_path_l] -> plot/3(qp_l)
  [dp_path_s_final] -> plot/1(dp_s)
  [dp_path_l_final] -> plot/2(dp_l)
  [l_min] -> plot/4(l_min)
  [l_max] -> plot/5(l_max)
  [plan_start_dl] -> plot/10(start_dl)
  [plan_start_l] -> plot/9(start_l)
  [plan_start_s] -> plot/8(start_s)
  [static_obs_s_set] -> plot/6(obs_s_set)
  [static_obs_l_set] -> plot/7(obs_l_set)
  path decision task/1(dp_path_s_final) -> [dp_path_s_final]
  path decision task/2(dp_path_l_final) -> [dp_path_l_final]
  path decision task/3(dp_path_dl_final) -> [dp_path_dl_final]
  path decision task/4(dp_path_ddl_final) -> [dp_path_ddl_final]
  [static_obs_s_set] -> path decision task/1(static_obs_s_set)
  [static_obs_l_set] -> path decision task/2(static_obs_l_set)
  [plan_start_ddl] -> path decision task/6(plan_start_ddl)
  [plan_start_dl] -> path decision task/5(plan_start_dl)
  [plan_start_l] -> path decision task/4(plan_start_l)
  [plan_start_s] -> path decision task/3(plan_start_s)
  path planning task/1(qp_path_l) -> [qp_path_l]
  path planning task/2(qp_path_dl) -> [qp_path_dl]
  path planning task/3(qp_path_ddl) -> [qp_path_ddl]
  [dp_path_s_final] -> path planning task/1(dp_path_s_final)
  [dp_path_l_final] -> path planning task/2(dp_path_l_final)
  [dp_path_dl_final] -> path planning task/3(static_obs_s_set)
  [dp_path_ddl_final] -> path planning task/4(static_obs_l_set)
  [plan_start_l] -> path planning task/5(plan_start_l)
  [plan_start_ddl] -> path planning task/7(plan_start_ddl)
  [plan_start_dl] -> path planning task/6(plan_start_dl)
  Constant22/1 -> path planning task/18(host_w)
  Constant21/1 -> path planning task/17(host_d2)
  Constant20/1 -> path planning task/16(host_d1)
  Constant19/1 -> path planning task/15(qp_cost_end_ddl)
  Constant18/1 -> path planning task/14(qp_cost_end_dl)
  Constant17/1 -> path planning task/13(qp_cost_endl)
  Constant16/1 -> path planning task/12(qp_cost_centre)
  Constant15/1 -> path planning task/11(qp_cost_dddl)
  Constant14/1 -> path planning task/10(qp_cost_ddl)
  Constant13/1 -> path planning task/9(qp_cost_dl)
  Constant12/1 -> path planning task/8(qp_cost_l)
  Constant8/1 -> path decision task/15(dp_sample_l)
  Constant7/1 -> path decision task/14(dp_sample_s)
  Constant6/1 -> path decision task/13(dp_col)
  Constant5/1 -> path decision task/12(dp_row)
  Constant4/1 -> path decision task/11(dp_cost_ref)
  Constant3/1 -> path decision task/10(dp_cost_dddl)
  Constant/1 -> path decision task/7(dp_cost_collision)
  Constant1/1 -> path decision task/8(dp_cost_dl)
  Constant2/1 -> path decision task/9(dp_cost_ddl)
